simulink model "ex4"  (R2020a)
settings: Solver=VariableStepAuto  StartTime=0.0  StopTime=10.0  RelTol=1e-3

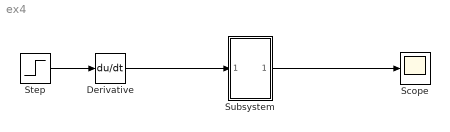
== system ex4 ==
  Derivative : Derivative
  Scope : Scope
  Step : Step  SampleTime=0.1
  Subsystem : Subsystem  mask{Te=0.1}
      mask prompts: Te "Te="
      mask Callback Te:
      | if str2num(get_param(gcb,'Te'))<0
      |     error('Perioada de esantionare negativa')
      | end
  wires:
  Step/1 -> Derivative/1
  Derivative/1 -> Subsystem/1(In1)
  Subsystem/1(Out1) -> Scope/1

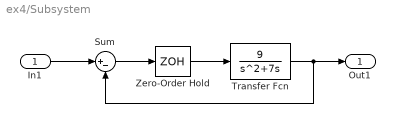
== system ex4/Subsystem ==
  In1 : Inport
  Sum : Sum  Inputs=|+-  SampleTime=Te
  Transfer Fcn : TransferFcn  Numerator=[9]  Denominator=[1 7 0]
  Zero-Order Hold : ZeroOrderHold  SampleTime=-1
  Out1 : Outport
  wires:
  Zero-Order Hold/1 -> Transfer Fcn/1
  Sum/1 -> Zero-Order Hold/1
  Transfer Fcn/1 -> Out1/1, Sum/2
  In1/1 -> Sum/1
